simulink model "get_smn_sfunc_output_dim"  (Simulink 6.3)
settings: Solver=FixedStepDiscrete  StartTime=0.0  StopTime=0.0  FixedStep=1  RelTol=1e-3
undefined symbols (not defined in the file or in its folder): MACH
settings Model: Creator=spratt  LastModifiedBy=spratt  ExtModeAutoUpdateStatusClock=off

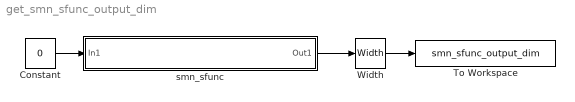
== system get_smn_sfunc_output_dim ==
  Constant : Constant  Value=0
  To Workspace : ToWorkspace  VariableName=smn_sfunc_output_dim  SampleTime=-1  SaveFormat=Array
  Width : Width
  smn_sfunc : Subsystem  mask{sfunc_name=MACH.smn_sfunc_name}
      mask prompts: sfunc_name "S-function name"
      mask init:
      | block_name = [gcb '/S-Function'];
      | % disp(sprintf('S-Function name = %s',sfunc_name))
      | try
      |     set_param(block_name,'FunctionName',sfunc_name);
      |     % disp(sprintf('setting %s to %s',block_name,sfunc_name));
      | % catch
      | %    set_param(block_name,'FunctionName','smn_sfunc');
      |     % disp(sprintf('setting %s to %s',block_name,'smn_sfunc'));
      | end
      mask Display: disp(sfunc_name)
  wires:
  Constant/1 -> smn_sfunc/1(In1)
  smn_sfunc/1(Out1) -> Width/1
  Width/1 -> To Workspace/1

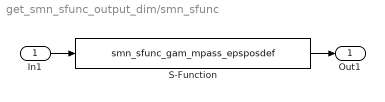
== system get_smn_sfunc_output_dim/smn_sfunc ==
  In1 : Inport
  S-Function : S-Function  FunctionName=smn_sfunc_gam_mpass_epsposdef
  Out1 : Outport
  wires:
  In1/1 -> S-Function/1
  S-Function/1 -> Out1/1
